simulink model "PandO_Model_basepaper"  (R2020a)
settings: Solver=VariableStepAuto  StartTime=0.0  StopTime=1  RelTol=1e-3
undefined symbols (not defined in the file or in its folder): sigbuilder_block
libraries: powerlib x12, powerlib_meascontrol x2, simulink x1, re_lib x1
settings Model: Creator=sameeraa  LastModifiedBy=sameeraa

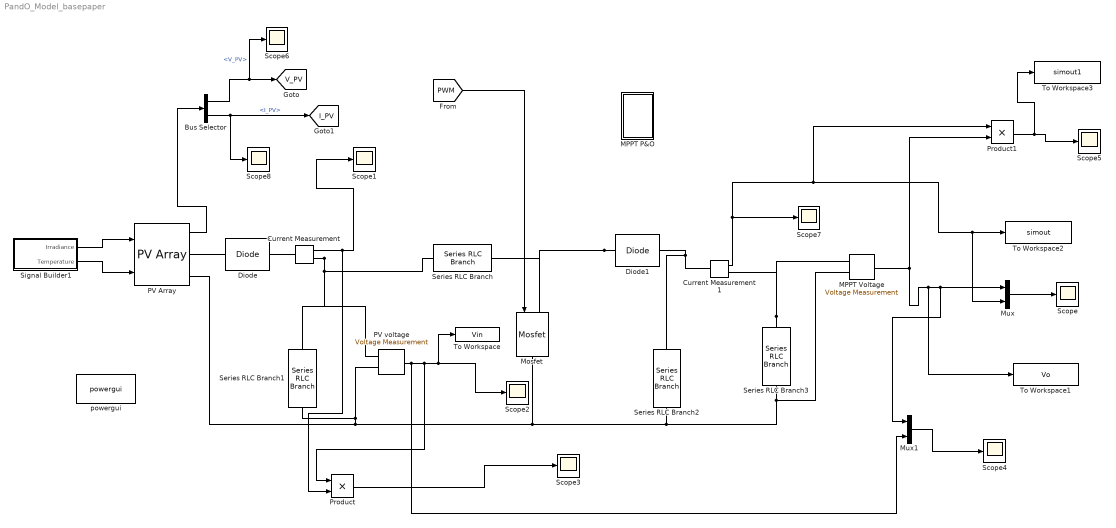
== system PandO_Model_basepaper ==
  Bus Selector : BusSelector  OutputSignals=V_PV,I_PV
  Current Measurement : powerlib/Measurements/Current Measurement  PhasorSimulation=off  OutputType=Complex  PSBequivalent=0
  Current Measurement1 : powerlib/Measurements/Current Measurement  PhasorSimulation=off  OutputType=Complex  PSBequivalent=0
  Diode : powerlib/Power Electronics/Diode  Ron=0.001  Lon=0  Vf=0.8  IC=0  UseSnubber=0  Rs=0  Cs=0  Measurements=off
  Diode1 : powerlib/Power Electronics/Diode  Ron=0.001  Lon=0  Vf=0.8  IC=0  UseSnubber=0  Rs=500  Cs=250e-9  Measurements=off
  MPPT P&O : Subsystem
  MPPT Voltage : powerlib/Measurements/Voltage Measurement  PhasorSimulation=off  OutputType=Complex  PSBequivalent=0
  Mosfet : powerlib/Power Electronics/Mosfet  Ron=0.1  Lon=0  Rd=0.01  Vfd=0  IC=0  Rs=1e5  Cs=inf  Measurements=off
  Mux : Mux  Inputs=2
  Mux1 : Mux  Inputs=2
  PV Array : re_lib/Solar/PV Array  Npar=1  Nser=1  PlotType=one module @ 25 deg.C & specified irradiances  S_vec="[ 1000  800  600 ]"  Temp_C_vec="[ 45 25  ]"  ModuleName=User-defined  PlotWhenSelected=off  Pm=223.3  Ncell=60  Voc=36.3  Isc=7.84  Vm=29  Im=7.7  beta_Voc_pc=-0.36099  alpha_Isc_pc=0.102  beta_Voc=-0.13104  alpha_Isc=0.0079968  IL=8.0515  I0=2.9406e-10  nI=0.97985  Rsh=6175.6519  Rs=0.38059  RobustModel=off  RobustCellTemperature=25  BAL=on  Tc=1e-6  Tfilter=5e-5
  PV voltage : powerlib/Measurements/Voltage Measurement  PhasorSimulation=off  OutputType=Complex  PSBequivalent=0
  Product : Product
  Product1 : Product
  Scope{,1..8} (9 alike) : Scope
  Series RLC Branch : powerlib/Elements/Series RLC Branch  LConnTagsString=__new0  RConnTagsString=__new0  BranchType=L  Resistance=1  Inductance=1e-3  SetiL0=off  InitialCurrent=0  Capacitance=1e-6  Setx0=off  InitialVoltage=0  Measurements=None
  Series RLC Branch1 : powerlib/Elements/Series RLC Branch  LConnTagsString=__new0  RConnTagsString=__new0  BranchType=C  Resistance=1  Inductance=1e-3  SetiL0=off  InitialCurrent=0  Capacitance=377e-6  Setx0=off  InitialVoltage=0  Measurements=None
  Series RLC Branch2 : powerlib/Elements/Series RLC Branch  LConnTagsString=__new0  RConnTagsString=__new0  BranchType=C  Resistance=1  Inductance=1e-3  SetiL0=off  InitialCurrent=0  Capacitance=377e-6  Setx0=off  InitialVoltage=0  Measurements=None
  Series RLC Branch3 : powerlib/Elements/Series RLC Branch  LConnTagsString=__new0  RConnTagsString=__new0  BranchType=R  Resistance=5  Inductance=1e-3  SetiL0=off  InitialCurrent=0  Capacitance=1e-6  Setx0=off  InitialVoltage=0  Measurements=None
  Signal Builder1 : Subsystem  Tag=STV Subsys  LoadFcn=sigbuilder_block('load');  StartFcn=sigbuilder_block('start');  StopFcn=sigbuilder_block('stop');  ClipboardFcn=sigbuilder_block('clipboard');  mask(Sigbuilder block){tuvar=[0:10]}
      mask help: Simulink:masks:SigbuilderBlock_MD
      mask init:
      | if ~strcmp(get_param(bdroot(gcbh),'SimulationStatus'),'stopped') tuvar = sigbuilder_block('maskInit'); end
      settings: CopyFcn=sigbuilder_block('copy');  DeleteFcn=sigbuilder_block('delete');  ModelCloseFcn=sigbuilder_block('modelClose');  PreSaveFcn=sigbuilder_block('preSave');  PauseFcn=sigbuilder_block('pause');  ContinueFcn=sigbuilder_block('continue');  NameChangeFcn=sigbuilder_block('namechange');  OpenFcn=sigbuilder_block('open',[382.8 123 550.8 400.2 ]);  CloseFcn=sigbuilder_block('close');
      mask Display: plot(0, 0, 100, 100,[2, 2, 32, 32, 2], [68, 8, 8, 68, 68],[32, 2], [38, 38], [32, 19, 2],[53, 60, 44], [32, 17, 17, 2],[16, 16, 31, 31]);txt = getActiveGroup(gcbh);text(2, 100, txt,'verticalAlignment', 'top');
  To Workspace : ToWorkspace  VariableName=Vin  SampleTime=-1
  To Workspace1 : ToWorkspace  VariableName=Vo  SampleTime=-1
  To Workspace2 : ToWorkspace  VariableName=simout  SaveFormat=Timeseries  SampleTime=-1
  To Workspace3 : ToWorkspace  VariableName=simout1  SaveFormat=Timeseries  SampleTime=-1
  powergui : powerlib/powergui  Priority=1  SimulationMode=Continuous  SampleTime=50e-6  frequency=60  Iterations=50  frequencyindice=0  Pbase=100e6  ErrMax=1e-4  UnitsV=kV  UnitsW=MW  buscounter=0  FunctionMessages=off  echomessages=off  EnableUseOfTLC=off  CurrentSourceSwitches=off  DisableSnubberDevices=off  DisableRonSwitches=off  DisableVfSwitches=off  DisplayEquations=off  AutomaticDiscreteSolvers=off  SolverType=Tustin/Backward Euler (TBE)  Interpol=off  ExternalGateDelay=off  methode=off  Ts=100  x0status=blocks  SPID=on  SwTol=0  HookPort=off  NonlinearTolerance=1e-4  nMaxIteration=100  ContinueOnMaxIteration=off  RestoreLinks=warning  ResistiveCurrentMeasurement=off  Frange=[0:2:500]  Ylog=off  Xlog=on  ShowGrid=off  save=off  variable=ZData  structure=0  ZoomFFT=off  StartTime=0.0  cycles=1  DisplayStyle=1  fundamental=60  FreqAxis=off  MaxFrequency=1000  frequencyindicesteady=1  RmsSteady=1  display=off
  tag scope: I_PV=global, V_PV=global
  wires:
  Signal Builder1/1(Irradiance) -> PV Array/1
  PV voltage/1 -> Scope2/1, To Workspace/1, Product/1, Mux1/2
  Bus Selector/1 -> Scope6/1, [V_PV]  "<V_PV>"
  PV Array/1 -> Bus Selector/1
  [PWM] -> Mosfet/1
  Bus Selector/2 -> [I_PV], Scope8/1  "<I_PV>"
  Mux/1 -> Scope/1
  Current Measurement1/1 -> Scope7/1, Product1/1, To Workspace2/1, Mux/2
  Signal Builder1/2(Temperature) -> PV Array/2
  Product1/1 -> To Workspace3/1, Scope5/1
  Product/1 -> Scope3/1
  Mux1/1 -> Scope4/1
  Current Measurement/1 -> Product/2, Scope1/1
  MPPT Voltage/1 -> To Workspace1/1, Mux/1, Mux1/1, Product1/2
  connections:
  Series RLC Branch3/RConn1 -- MPPT Voltage/LConn2 -- Series RLC Branch2/RConn1 -- PV Array/RConn2 -- PV voltage/LConn2 -- Series RLC Branch1/RConn1 -- Mosfet/RConn1
  Current Measurement/RConn1 -- Series RLC Branch1/LConn1 -- PV voltage/LConn1 -- Series RLC Branch/LConn1
  Series RLC Branch2/LConn1 -- Current Measurement1/LConn1 -- Diode1/RConn1
  Series RLC Branch3/LConn1 -- MPPT Voltage/LConn1 -- Current Measurement1/RConn1
  Diode1/LConn1 -- Mosfet/LConn1 -- Series RLC Branch/RConn1
  Diode/RConn1 -- Current Measurement/LConn1
  PV Array/RConn1 -- Diode/LConn1

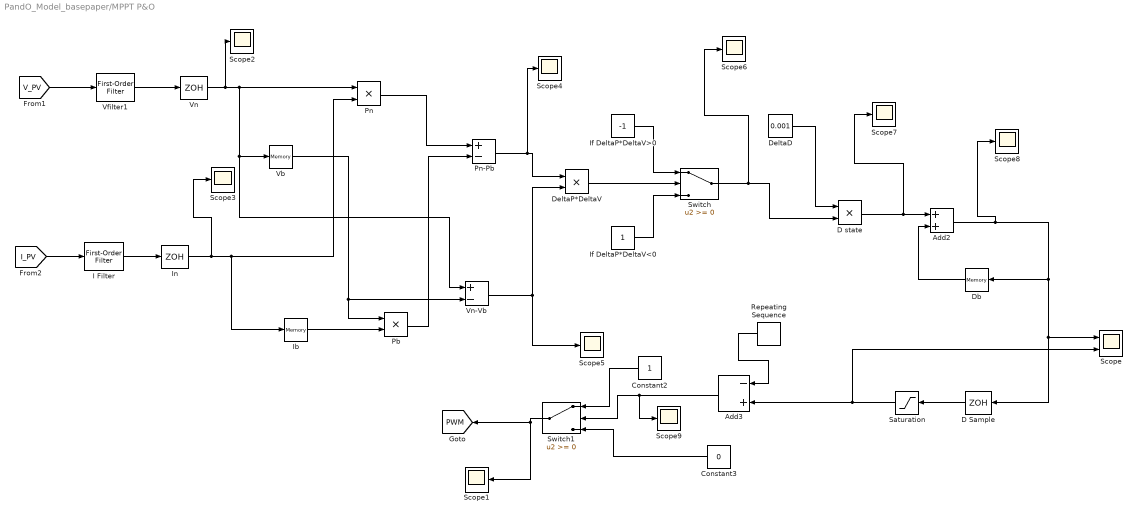
== system PandO_Model_basepaper/MPPT P&O ==
  Add2 : Sum
  Add3 : Sum  Inputs=-+
  Constant2 : Constant
  Constant3 : Constant  Value=0
  D Sample : ZeroOrderHold  SampleTime=-1
  D state : Product
  Db : Memory
  DeltaD : Constant  Value=0.001
  DeltaP*DeltaV : Product
  I Filter : powerlib_meascontrol/Filters/First-Order Filter  FilterType=Lowpass  Tc=10e-3  Ts=0  Initialize=on  Vac_Init=[0, 0, 60]  Vdc_Init=0  PlotResponse=off  FreqRange="[0,  200,  1]"
  Ib : Memory
  If DeltaP*DeltaV<0 : Constant
  If DeltaP*DeltaV>0 : Constant  Value=-1
  In : ZeroOrderHold  SampleTime=-1
  Pb : Product
  Pn : Product
  Pn-Pb : Sum  Inputs=+-
  Repeating Sequence : simulink/Sources/Repeating Sequence  rep_seq_t=[0 0.02]  rep_seq_y=[0 2]
  Saturation : Saturate
  Scope : Scope  NumInputPorts=2
  Scope{1..9} (9 alike) : Scope
  Switch : Switch
  Switch1 : Switch
  Vb : Memory
  Vfilter1 : powerlib_meascontrol/Filters/First-Order Filter  FilterType=Lowpass  Tc=10e-3  Ts=0  Initialize=on  Vac_Init=[0, 0, 60]  Vdc_Init=0  PlotResponse=off  FreqRange="[0,  200,  1]"
  Vn : ZeroOrderHold  SampleTime=-1
  Vn-Vb : Sum  Inputs=+-
  tag scope: PWM=global
  wires:
  Vn-Vb/1 -> DeltaP*DeltaV/2, Scope5/1
  Ib/1 -> Pb/2
  Vn/1 -> Scope2/1, Vn-Vb/1, Vb/1, Pn/1
  Pn-Pb/1 -> Scope4/1, DeltaP*DeltaV/1
  Add2/1 -> Scope8/1, Db/1, Scope/1, D Sample/1
  D Sample/1 -> Saturation/1
  Constant3/1 -> Switch1/3
  Pn/1 -> Pn-Pb/1
  Switch/1 -> Scope6/1, D state/2
  Pb/1 -> Pn-Pb/2
  Db/1 -> Add2/2
  D state/1 -> Scope7/1, Add2/1
  DeltaP*DeltaV/1 -> Switch/2
  If DeltaP*DeltaV>0/1 -> Switch/1
  If DeltaP*DeltaV<0/1 -> Switch/3
  Switch1/1 -> Scope1/1, [PWM]
  Vb/1 -> Pb/1, Vn-Vb/2
  Constant2/1 -> Switch1/1
  Repeating Sequence/1 -> Add3/1
  Add3/1 -> Scope9/1, Switch1/2
  In/1 -> Scope3/1, Ib/1, Pn/2
  DeltaD/1 -> D state/1
  [I_PV] -> I Filter/1
  [V_PV] -> Vfilter1/1
  Saturation/1 -> Scope/2, Add3/2
  Vfilter1/1 -> Vn/1
  I Filter/1 -> In/1

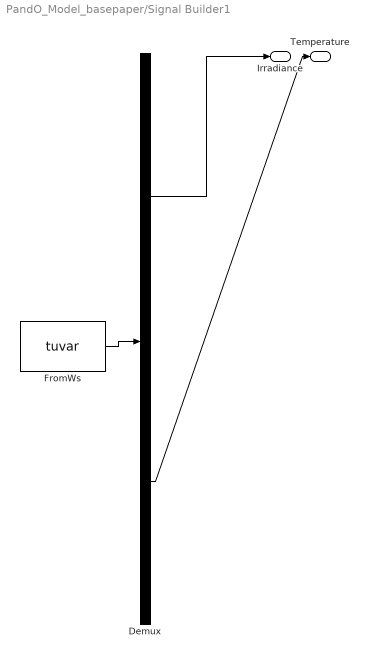
== system PandO_Model_basepaper/Signal Builder1 ==
  Demux : Demux  Tag=STV Demux  Outputs=2
      settings: DisplayOption=none
  FromWs : FromWorkspace  Tag=STV FromWs  VariableName=tuvar
      SigBuilderData=|
      | common.afterFinalStr = 'Extrapolate'
      | common.sampleTime = 0
      | dataSet.timeRange = [0 10]
      | dataSet.name = 'Group 1'
      | sbobj.Groups.Name = 'Group 1'
      | sbobj.Groups.Signals(1).Name = 'Irradiance'
      | sbobj.Groups.Signals(1).XData = [0 10]
      | sbobj.Groups.Signals(1).YData = [1000 1000]
      | sbobj.Groups.Signals(2).Name = 'Temperature'
      | sbobj.Groups.Signals(2).XData = [0 10]
      | sbobj.Groups.Signals(2).YData = [25 25]
  Irradiance : Outport  Tag=STV Outport
  Temperature : Outport  Tag=STV Outport  Port=2
  wires:
  Demux/1 -> Irradiance/1
  FromWs/1 -> Demux/1
  Demux/2 -> Temperature/1
